simulink model "test_01"  (R2018a)
settings: Solver=FixedStepDiscrete  StartTime=0.0  StopTime=60  FixedStep=0.01  RelTol=1e-3
undefined symbols (not defined in the file): DiscIntNeverNeededParam, histPoints
libraries: dspsrcs4 x5, sldrtlib x1
settings Model: Creator=lichaoqun  LastModifiedBy=lichaoqun
settings OptimizationCC: DefaultParameterBehavior=Inlined  EnhancedBackFolding=on  PassReuseOutputArgsAs=Individual arguments  OptimizeBlockOrder=speed  DifferentSizesBufferReuse=on  OptimizationCustomize=off
settings DebuggingCC: ParameterTunabilityLossMsg=error
settings SFSimCC: MATLABDynamicMemAlloc=off
settings RTWCC: SystemTargetFile=ert.tlc  TemplateMakefile=ert_default_tmf  GenerateReport=on  IncludeHyperlinkInReport=on  LaunchReport=on  GenerateTraceInfo=on  GenerateTraceReport=on  GenerateTraceReportSl=on  GenerateTraceReportSf=on  GenerateTraceReportEml=on
settings CodeAppCC: ForceParamTrailComments=on  IgnoreCustomStorageClasses=off  OperatorAnnotations=on  SimulinkDataObjDesc=on  SFDataObjDesc=on  InsertBlockDesc=on
settings ERTTargetCC: TargetLangStandard=C99 (ISO)  GenerateSampleERTMain=on  InlinedParameterPlacement=NonHierarchical  ERTCustomFileTemplate=example_file_process.tlc

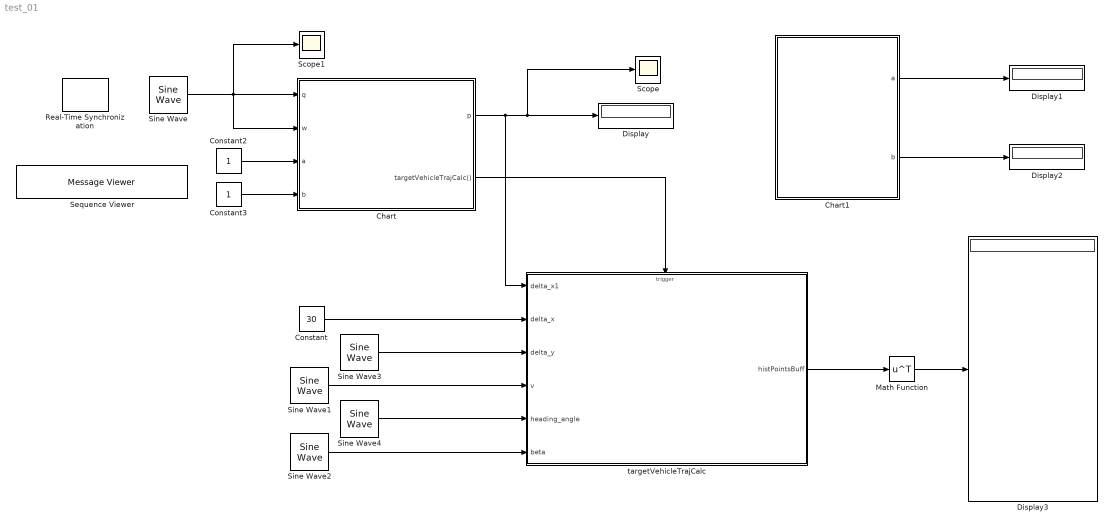
== system test_01 ==
  Chart : Stateflow chart  TreatAsAtomicUnit=on
  Chart1 : Stateflow chart  TreatAsAtomicUnit=on
  Constant : Constant  Value=30
  Constant2 : Constant
  Constant3 : Constant
  Display{,1..3} (4 alike) : Display
  Math Function : Math  Operator=transpose  SaturateOnIntegerOverflow=on
  Real-Time Synchronization : sldrtlib/Real-Time Synchronization  SampleTime=0.1  MaxMissedTicks=100  ShowMissedTicks=off  YieldWhenWaiting=off
  Scope : Scope
  Scope1 : Scope
  Sequence Viewer : MessageViewer
  Sine Wave : dspsrcs4/Sine Wave  Amplitude=1  Frequency=0.1  Phase=0  SampleMode=Discrete  OutComplex=Real  CompMethod=Trigonometric fcn  TableSize=Speed  SampleTime=0.01  SamplesPerFrame=1  ResetState=Restart at time zero  OutputFrames=off  dataType=double  wordLen=16  udDataType=sfix(16)  fracBitsMode=Best precision  numFracBits=15  OutDataTypeStr=double  LastOutDataTypeStr=double
  Sine Wave1 : dspsrcs4/Sine Wave  Amplitude=10  Frequency=0.1  Phase=0  SampleMode=Discrete  OutComplex=Real  CompMethod=Trigonometric fcn  TableSize=Speed  SampleTime=0.01  SamplesPerFrame=1  ResetState=Restart at time zero  OutputFrames=off  dataType=double  wordLen=16  udDataType=sfix(16)  fracBitsMode=Best precision  numFracBits=15  OutDataTypeStr=double  LastOutDataTypeStr=double
  Sine Wave2 : dspsrcs4/Sine Wave  Amplitude=1  Frequency=0.1  Phase=0  SampleMode=Discrete  OutComplex=Real  CompMethod=Trigonometric fcn  TableSize=Speed  SampleTime=0.01  SamplesPerFrame=1  ResetState=Restart at time zero  OutputFrames=off  dataType=double  wordLen=16  udDataType=sfix(16)  fracBitsMode=Best precision  numFracBits=15  OutDataTypeStr=double  LastOutDataTypeStr=double
  Sine Wave3 : dspsrcs4/Sine Wave  Amplitude=3  Frequency=0.1  Phase=0  SampleMode=Discrete  OutComplex=Real  CompMethod=Trigonometric fcn  TableSize=Speed  SampleTime=0.01  SamplesPerFrame=1  ResetState=Restart at time zero  OutputFrames=off  dataType=double  wordLen=16  udDataType=sfix(16)  fracBitsMode=Best precision  numFracBits=15  OutDataTypeStr=double  LastOutDataTypeStr=double
  Sine Wave4 : dspsrcs4/Sine Wave  Amplitude=1  Frequency=0.1  Phase=0  SampleMode=Discrete  OutComplex=Real  CompMethod=Trigonometric fcn  TableSize=Speed  SampleTime=0.01  SamplesPerFrame=1  ResetState=Restart at time zero  OutputFrames=off  dataType=double  wordLen=16  udDataType=sfix(16)  fracBitsMode=Best precision  numFracBits=15  OutDataTypeStr=double  LastOutDataTypeStr=double
  targetVehicleTrajCalc : Subsystem  TreatAsAtomicUnit=on
      settings: RTWFcnNameOpts=Use subsystem name  RTWFileNameOpts=Use subsystem name
  wires:
  Sine Wave/1 -> Scope1/1, Chart/2(w), Chart/1(q)
  Chart/1(p) -> Display/1, Scope/1, targetVehicleTrajCalc/1(delta_x1)
  Constant2/1 -> Chart/3(a)
  Constant3/1 -> Chart/4(b)
  Chart1/1(a) -> Display1/1
  Chart1/2(b) -> Display2/1
  Sine Wave1/1 -> targetVehicleTrajCalc/4(v)
  Sine Wave4/1 -> targetVehicleTrajCalc/5(heading_angle)
  Sine Wave2/1 -> targetVehicleTrajCalc/6(beta)
  Constant/1 -> targetVehicleTrajCalc/2(delta_x)
  Sine Wave3/1 -> targetVehicleTrajCalc/3(delta_y)
  targetVehicleTrajCalc/1(histPointsBuff) -> Math Function/1
  Math Function/1 -> Display3/1
  Chart/2(targetVehicleTrajCalc()) -> targetVehicleTrajCalc/Trigger

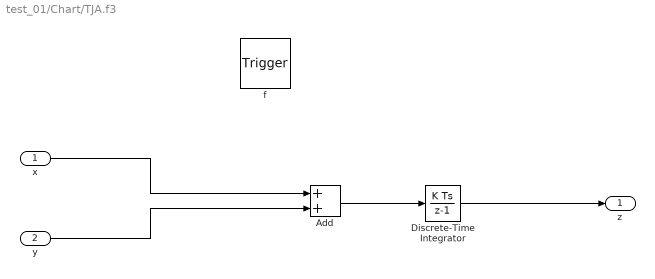
== system test_01/Chart/TJA.f3 ==
  x : Inport  OutDataTypeStr=double  PortDimensions=1
  y : Inport  Port=2  OutDataTypeStr=double  PortDimensions=1
  f : TriggerPort  TriggerType=function-call  VariantControl=(inherit)
      settings: CopyFcn=Stateflow.SLINSF.SimulinkMan.removeBlockPreDeleteFcn  PreDeleteFcn=Stateflow.SLINSF.SimulinkMan.unsafePredeleteFcn
  Add : Sum
  Discrete-Time Integrator : DiscreteIntegrator  SampleTime=-1  ICPrevOutput=DiscIntNeverNeededParam  ICPrevScaledInput=DiscIntNeverNeededParam
  z : Outport  OutDataTypeStr=double  PortDimensions=1
  wires:
  y/1 -> Add/2
  x/1 -> Add/1
  Add/1 -> Discrete-Time Integrator/1
  Discrete-Time Integrator/1 -> z/1

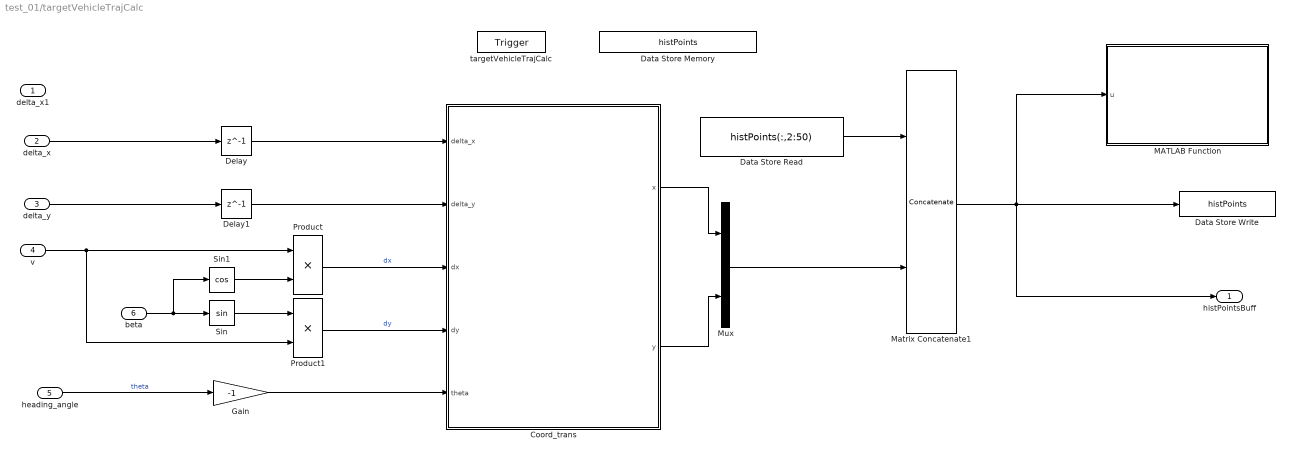
== system test_01/targetVehicleTrajCalc ==
  delta_x1 : Inport
  delta_x : Inport  Port=2
  delta_y : Inport  Port=3
  v : Inport  Port=4
  heading_angle : Inport  Port=5
  beta : Inport  Port=6
  targetVehicleTrajCalc : TriggerPort  TriggerType=function-call  VariantControl=Variant
  Coord_trans : MATLAB Function  TreatAsAtomicUnit=on
  Data Store Memory : DataStoreMemory  DataStoreName=histPoints  ReadBeforeWriteMsg=warning  WriteAfterWriteMsg=warning  WriteAfterReadMsg=warning  ShowAdditionalParam=off  Dimensions=[2 50]
  Data Store Read : DataStoreRead  DataStoreName=histPoints  DataStoreElements=histPoints(:,2:50)
  Data Store Write : DataStoreWrite  DataStoreName=histPoints
  Delay : Delay  DelayLength=1
  Delay1 : Delay  DelayLength=1
  Gain : Gain  Gain=-1
  MATLAB Function : MATLAB Function  TreatAsAtomicUnit=on
  Matrix Concatenate1 : Concatenate  Mode=Multidimensional array  ConcatenateDimension=2
  Mux : Mux  Inputs=2
  Product : Product
  Product1 : Product
  Sin : Trigonometry
  Sin1 : Trigonometry  Operator=cos
  histPointsBuff : Outport
  wires:
  beta/1 -> Sin1/1, Sin/1
  Sin1/1 -> Product/2
  v/1 -> Product/1, Product1/2
  Sin/1 -> Product1/1
  Product/1 -> Coord_trans/3(dx)  "dx"
  Product1/1 -> Coord_trans/4(dy)  "dy"
  delta_x/1 -> Delay/1
  delta_y/1 -> Delay1/1
  Delay1/1 -> Coord_trans/2(delta_y)
  Delay/1 -> Coord_trans/1(delta_x)
  heading_angle/1 -> Gain/1  "theta"
  Data Store Read/1 -> Matrix Concatenate1/1
  Mux/1 -> Matrix Concatenate1/2
  Coord_trans/1(x) -> Mux/1
  Coord_trans/2(y) -> Mux/2
  Matrix Concatenate1/1 -> histPointsBuff/1, MATLAB Function/1(u), Data Store Write/1
  Gain/1 -> Coord_trans/5(theta)

== stateflow chart test_01/Chart1 ==
  state A
    en:
    a=1;
    du:
    a=2;
    exit:
    a=3;
    state A1
    state A2
    (default) -> A1
    A1 -> A2 : after(0.01,sec)
  state B
    (default) -> (junction 25)
    (junction 25) -> (junction 24) : {b++}
  (default) -> A
  A -> B : after(0.02,sec)
  B -> A : after(0.02,sec)
  data: a output; b output double

== matlab function test_01/targetVehicleTrajCalc/Coord_trans ==
  data: x output; delta_x input; y output; delta_y input; dx input; dy input; theta input
function [x, y] = fcn(delta_x, delta_y, dx, dy, theta)
x = (delta_x - dx)*cos(theta) + (delta_y - dy)*sin(theta);
y = (delta_y - dy)*cos(theta) -  (delta_x - dx)*sin(theta);

== stateflow chart test_01/Chart ==
  state TJA [group]
    state OFF
      state B [parallel]
        settings: executionOrder=1
        (default) -> (junction 24)
        (junction 24) -> (junction 26)
        (junction 26) -> (junction 28)
        (junction 28) -> (junction 30)
      state C [parallel]
        du:p = f3(q,w);
        settings: executionOrder=2
    state ON
      du:
      f1();
      send(targetVehicleTrajCalc);
    state FAIL
      du:f2()
    state f1 [function]
      (default) -> (junction 53)
      (junction 53) -> (junction 57) [order 1]
      (junction 57) -> (junction 59) [order 1]
      (junction 59) -> (junction 61)
      (junction 57) -> (junction 61) [order 2]
      (junction 53) -> (junction 61) [order 2]
    state z = f3(x,y) [function]
    (default) -> OFF
    (junction 42) -> OFF : after(2,sec)
    FAIL -> (junction 42)
    OFF -> ON : after(2,sec)
    ON -> FAIL : after(2,sec)
  data: x function_input double size=1; y function_input double size=1; z function_output double size=1; p output; q input; w input; a input; b input
  events: targetVehicleTrajCalc output FUNCTION_CALL_EVENT
  function f2:
    | function f2

== matlab function test_01/targetVehicleTrajCalc/MATLAB Function ==
  data: u input
function plotTraj(u)
N = 50;
X = u(1,:);
Y = u(2,:);

p=polyfit(X, Y,3);  

xi=linspace(X(1), X(50),50);

yi=polyval(p,xi);  

plot(xi,yi, 'r', X, Y, 'b');
